simulink library "pwrsys"  (R2018a)
settings: Solver=VariableStepAuto  StartTime=0.0  StopTime=10.0  RelTol=1e-3
values from neighbouring files (symbols this model uses):
  Ts = Ts_c    (= 1e-07)    [PlantStateEquations_abc_Script.m]
undefined symbols (not defined in the file or in its folder): D1, Delta, DiscIntNeverNeededParam, ESS, f_LPF_noise, fn, fsw, grid, gt1, Iap, Kp, PCC, Refmax, Refmin, sim, SIMU, Sn, tctrl, Ti, Ts_control, Ts_PWM, Uabp, Uanp, WT, X, zeta
libraries: $bdroot x71, powerlib x59, powerlib_meascontrol x49, peTransforms x20, PhD_Library x1, sps_avr x1
(part 1 of 4)
settings Model: Creator=daniemot  LastModifiedBy=ericfa

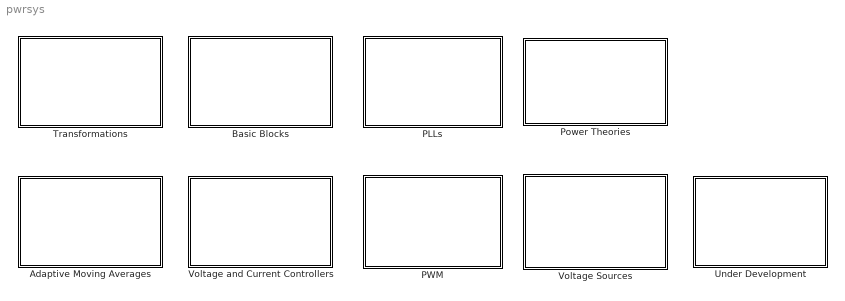
== system pwrsys ==
  Adaptive Moving Averages : Subsystem
  Basic Blocks : Subsystem
  PLLs : Subsystem
  PWM : Subsystem
  Power Theories : Subsystem
  Transformations : Subsystem
  Under Development : Subsystem
  Voltage Sources : Subsystem
  Voltage and Current Controllers : Subsystem

== system pwrsys/Adaptive Moving Averages ==
  AMA with insertion pointer driven buffer : Subsystem  TreatAsAtomicUnit=on  SystemSampleTime=Ts  mask(AMA with insertion pointer driven){NbSize=100, Ts=0.001}
      mask prompts: NbSize "Max number of samples for averaging"; Ts "Sampling time [s]"
      mask help:
      | Adaptive moving average with insertion pointer driven circular buffer
      |
      | Interface
      | Input	x (scalar): signal for averaging
      | 	n (scalar): number of previous samples of the input to be averaged with the current input
      | Output	xavg (scalar): average of the current input and the last n-samples of the input.
      | 	xacc (scalar): internal value sent for accumulation
      | 	xdec (scalar): internal value sent for decumulation
      | Parameters	nmax (scalar): maximum length of the length of the circular buffer
      | 	Ts (scalar): sampling time in [s]
      | Internal circular buffer:
      | 	Insertion pointer: i, always marches forward, x(now) replaces the slot pointed by i
      | 	Retrieval pointer: r, lags i by n samples, zeros the slot once retrieved, allowed to jump backwards, collects all values for decumulation and zeros slots when jumping forward.
      |
      | Prog/rev. semi-history:
      | 	Mota, 2020-11-24: first release
  AMA with lossy buffer : Subsystem  TreatAsAtomicUnit=on  SystemSampleTime=Ts  mask(AMA with a skipping circular buffer.){NbSize=100, Ts=0.001}
      mask prompts: NbSize "Max number of samples for averaging"; Ts "Sampling time [s]"
      mask help:
      | Adaptive moving average built with Matlab's discrete variable time delay
      |
      | Interface
      | Input	x (scalar): signal for averaging
      | 	n (scalar): number of previous samples of the input to be averaged with the current input
      | Output	xavg (scalar): average of the current input and the last n-samples of the input.
      | 	xacc (scalar): internal value sent for accumulation
      | 	xdec (scalar): internal value sent for decumulation
      | Parameters	nmax (scalar): maximum length of the length of the circular buffer
      | 	Ts (scalar): sampling time in [s]
      | Internal circular buffer:
      | 	Matlab's variable discrete time delay
      | 	Skips/double decumulations when n changes
      |
      | Prog/rev. semi-history:
      | 	Mota, 2020-11-24: first release
  AMA with retrieval pointer driven buffer : Subsystem  TreatAsAtomicUnit=on  SystemSampleTime=Ts  mask(AMA with retrieval pointer driven buffer){NbSize=100, Ts=0.001}
      mask prompts: NbSize "Max number of samples for averaging"; Ts "Sampling time [s]"
      mask help:
      | Adaptive moving average with retrieval poitner driven circular buffer
      |
      | Interface
      | Input	x (scalar): signal for averaging
      | 	n (scalar): number of previous samples of the input to be averaged with the current input
      | Output	xavg (scalar): average of the current input and the last n-samples of the input.
      | 	xacc (scalar): internal value sent for accumulation
      | 	xdec (scalar): internal value sent for decumulation
      | Parameters	nmax (scalar): maximum length of the length of the circular buffer
      | 	Ts (scalar): sampling time in [s]
      | Internal circular buffer:
      | 	Retrieval pointer: r, always marches forward, zero the slot after retrieval.
      | 	Insertion pointer: i, marches n slots ahead of r, allowed to jump, sums x(now) to the whichever value present at the insertion slot
      |
      | Prog/rev. semi-history:
      | 	Mota, 2020-11-24: first release
  Subsystem : Subsystem  TreatAsAtomicUnit=on  SystemSampleTime=Ts  mask(HAMA with retrieval pointer driven buffer){NbSize=100, Ts=0.001}
      mask prompts: NbSize "Max number of samples for averaging"; Ts "Sampling time [s]"
      mask help:
      | Hybrid adaptive moving average with three retrieval pointer driven circular buffers.
      |
      | Interface
      | Input	x (scalar): signal for averaging
      | 	n (scalar): number of previous samples of the input to be averaged with the current input
      | Output	xavg (scalar): average of the current input and the last hybrid number of 'n'-samples of the input.
      | 	xavground (scalar): average of the current input and the last round(n)-samples of the input.
      | 	xavgceil (scalar): average of the current input and the last ceil(n)-samples of the input.
      | 	xavgfloor (scalar): average of the current input and the last floor(n)-samples of the input.
      | 	xavgweighed (scalar): average of the current input and the last weighted(n)-samples of the input.
      | Parameters	nmax (scalar): maximum length of the length of the circular buffer
      | 	Ts (scalar): sampling time in [s]
      |
      | Prog/rev. semi-history:
      | 	Mota, 2020-12-08: first release
  WAMA with insertion pointer driven buffer : Subsystem  TreatAsAtomicUnit=on  SystemSampleTime=Ts  mask(WAMA with insertion pointer driven buffer){NbSize=0, Ts=0}
      mask prompts: NbSize "Max number of samples for averaging"; Ts "Sampling time [s]"
      mask help:
      | Adaptive moving average with two insertion pointer driven circular buffers.
      |
      | Interface
      | Input	x (scalar): signal for averaging
      | 	n (scalar): number of previous samples of the input to be averaged with the current input
      | Output	xavg (scalar): weigthed average of the current input and the last 'n'-samples of the input.
      | 	xavgceil (scalar): average of the current input and the last ceil(n)-samples of the input.
      | 	xavgfloor (scalar): average of the current input and the last floor(n)-samples of the input.
      | Parameters	nmax (scalar): maximum length of the length of the circular buffer
      | 	Ts (scalar): sampling time in [s]
      |
      | Prog/rev. semi-history:
      | 	Mota, 2020-11-24: first release
  WAMA with retrieval pointer driven buffers : Subsystem  TreatAsAtomicUnit=on  SystemSampleTime=Ts  mask(WAMA with retrieval pointer driven buffer){NbSize=100, Ts=0.001}
      mask prompts: NbSize "Max number of samples for averaging"; Ts "Sampling time [s]"
      mask help:
      | Adaptive moving average with two retrieval pointer driven circular buffers.
      |
      | Interface
      | Input	x (scalar): signal for averaging
      | 	n (scalar): number of previous samples of the input to be averaged with the current input
      | Output	xavg (scalar): weigthed average of the current input and the last 'n'-samples of the input.
      | 	xavgceil (scalar): average of the current input and the last ceil(n)-samples of the input.
      | 	xavgfloor (scalar): average of the current input and the last floor(n)-samples of the input.
      | Parameters	nmax (scalar): maximum length of the length of the circular buffer
      | 	Ts (scalar): sampling time in [s]
      |
      | Prog/rev. semi-history:
      | 	Mota, 2020-11-24: first release

== system pwrsys/Basic Blocks ==
  DSC : Subsystem
  "DSC Power " : Subsystem
  Digital first order LPF : Subsystem  mask(Digital first-order low-pass filter){Ts=tctrl, fcutout=fn/2^0.5}
      mask prompts: Ts "Sample times [s]"; fcutout "Cutout frequency [Hz]"
      mask help:
      | Continuous time transfer function:  1/(1 + s T)
      | 	where T [s] = 1 / (2 pi fcutout [Hz]).
      |
      | Actual digital transfer function:   alpha / (1 + ( alpha -1) z^{-1} )
      | 	with eq. of diffs.: y = alpha x + (1 - alpha) y z^{-1}
      | 	where alpha = Ts / ( 1/(2 pi fcutout) + Ts)
      mask Display: fprintf('1/(1+sT)');
  Droop controller : Subsystem  mask(Droop controller){Refmax=1, Refmin=-1, Ts=-1, Kp=1, Kd=0, Tr=0.1, flp=100, DB=0}
      mask prompts: Refmax "Max reference"; Refmin "Min reference"; Ts "Sample time"; Kp "Permanent gain"; Kd "Transient gain"; Tr "Reset time [s]"; flp "Low-pass filter cut-off frequency [Hz]"; DB "Dead-band"
      mask help:
      | This block implements a droop controller, i.e. it provides compensation of the input Ref based on the input Delta and Comp.
      |
      | The input Delta is used as input of a PD controller which provides permanent (proportional) and transient (derivative) droop of the input Ref.
      |
      | The input Comp divides the output value of the droop controller and may be used for other types of compensation.
      mask DialogControl DescGroupVar Prompt: Active Power and Frequency Controller
      mask DialogControl DescTextVar Prompt: This block implements a simplified model for power control with droop influence. It can be used either for active power with frequency droop influence or reactive power with voltage droop influence.
      mask DialogControl droop Prompt: Droop control
      mask DialogControl meas Prompt: Delta
  PI controller with Hold : Subsystem  mask(PI controller with anti-windup){Kp=1, Ki=0, Max=1, Min=-1, x0=0, Ts=1e-4}
      mask prompts: Kp "Proportional gain"; Ki "Integral gain"; Max "Maximum output"; Min "Minimum output"; x0 "Initial condition"; Ts "Sampling time"
      mask help:
      | This block implements a PI controller with anti-windup
      |
      | The input hold freezes the integrator and allows implementing anti-windup in control loops with feed-forward or dynamic limits
  PI_Kg_Kp_Ti_AntiWindup : Subsystem  TreatAsAtomicUnit=on  SystemSampleTime=Ts  mask(PI regulator with anti-windup){Ts=0.001, Kg=1, Kp=1, Ti=1, PI_max=1, PI_min=-1}
      mask prompts: Ts "Sampling time [s]"; Kg "Loop gain: Kg [pu]"; Kp "Proportional gain: Kp [pu]"; Ti "Integral time: Ti [s]"; PI_max "Maximum output [pu]"; PI_min "Minimum output [pu]"
      mask help:
      | Discrete PI regulator with forward Euler approximation for the integrator.
      |
      | Transfer function:
      | 	Kg (Kp + 1/sTi)
      |
      | The anti-windup freezes the integrator if the unlimited output of the PI goes beyond the limits.
      |
      | It is possible to disable the proportional (Kp) contribution.
      mask Display: fprintf('Kg(Kp+1/(sTi))');
  PI_Kp_Ti_AntiWindup : Subsystem  TreatAsAtomicUnit=on  SystemSampleTime=Ts  mask(PI regulator with anti-windup){Ts=0.001, Kp=10, Ti=1, PI_max=1, PI_min=-1}
      mask prompts: Ts "Sampling time [s]"; Kp "Proportional gain: Kp [pu]"; Ti "Integral time: Ti [s]"; PI_max "Maximum output [pu]"; PI_min "Minimum output [pu]"
      mask help:
      | Discrete PI regulator with forward Euler approximation for the integrator.
      |
      | Transfer function:
      | 	Kp (1 + sTi) / (sTi)
      |
      | The anti-windup freezes the integrator if the unlimited output of the PI goes beyond the limits.
      mask Display: fprintf('Kp(1+1/(sTi))');
  PQVI : Subsystem  mask(u i p q transducer - No zero sequence){Sn=Sn, Uanp=Uanp, Iap=Iap}
      mask prompts: Sn "Rated three-phase apparent power [VA]"; Uanp "Rated peak phase-to-groud voltage [V]"; Iap "Rated peak line current [A]"
      mask help:
      | Loosely based on Akagi 1984, but with Clarke Transformation for both the current and voltage
      | 	v  = (valpha^2 + vbeta^2)^0.5 / V_phase_peak
      | 	i   = (ialpha^2 + ibeta^2)^0.5 / I_line_peak
      | 	p  = 3/2 * (valpha ialpha +vbeta ibeta) / Sn
      | 	q  = 3/2 * (-valpha ibeta +vbeta ialpha) / Sn
  digital_integrator : Subsystem  SystemSampleTime=Ts  mask(Digital integrator){Ts=tctrl}
      mask prompts: Ts "Sample times [s]"
      mask Display: fprintf('1/s');
  digital_ramp_gen : Subsystem  SystemSampleTime=Ts  mask(Digital ramp generator){Ts=tctrl}
      mask prompts: Ts "Sample times [s]"
      mask help: Allways starts at zero. Can be forced to a value, and will stay there, but in the first two cycles will stay at zero.
      mask Display: fprintf('Ramp');
  pqui_Transd_DSC : Subsystem  mask(DSC u i p q transducer - No zero sequence){Ts=0.000005, fn=50, Sn=Sn, Uanp=Uanp, Iap=Iap}
      mask prompts: Ts "Sampling time [s]"; fn "Rated frequency [Hz]"; Sn "Rated three-phase apparent power [VA]"; Uanp "Rated peak phase-to-groud voltage [V]"; Iap "Rated peak line current [A]"
      mask help:
      | Loosely based on Akagi 1984, but with Clarke Transformation for both the current and voltage
      | 	v  = (valpha^2 + vbeta^2)^0.5 / V_phase_peak
      | 	i   = (ialpha^2 + ibeta^2)^0.5 / I_line_peak
      | 	p  = 3/2 * (valpha ialpha +vbeta ibeta) / Sn
      | 	q  = 3/2 * (-valpha ibeta +vbeta ialpha) / Sn
  pqui_Transd_NoZeroSeq : Subsystem  mask(u i p q transducer - No zero sequence){Sn=Sn, Uanp=Uanp, Iap=Iap}
      mask prompts: Sn "Rated three-phase apparent power [VA]"; Uanp "Rated peak phase-to-groud voltage [V]"; Iap "Rated peak line current [A]"
      mask help:
      | Loosely based on Akagi 1984, but with Clarke Transformation for both the current and voltage
      | 	v  = (valpha^2 + vbeta^2)^0.5 / V_phase_peak
      | 	i   = (ialpha^2 + ibeta^2)^0.5 / I_line_peak
      | 	p  = 3/2 * (valpha ialpha +vbeta ibeta) / Sn
      | 	q  = 3/2 * (-valpha ibeta +vbeta ialpha) / Sn
  pqui_Transd_NoZeroSeq_Filter : Subsystem  mask(u i p q transducer - No zero sequence){Ts=0.001, Sn=1000, fn=50, Uanp=1000, Iap=1000, fcutoutvi=1000, fcutoutpq=1000, zeta=0.7}
      mask prompts: Ts "Sampling time [s]"; Sn "Rated three-phase apparent power [VA]"; fn "Rated frequency [Hz]"; Uanp "Rated peak phase-to-groud voltage [V]"; Iap "Rated peak line current [A]"; fcutoutvi "Cutout freq. low-pass for v&i meas. [Hz]"; fcutoutpq "Cutout freq. low-pass for p&q meas. [Hz]"; zeta "Zeta for all second order filters"
      mask help:
      | Loosely based on Akagi 1984, but with Clarke Transformation for both the current and voltage
      | 	v  = (valpha^2 + vbeta^2)^0.5 / V_phase_peak
      | 	i   = (ialpha^2 + ibeta^2)^0.5 / I_line_peak
      | 	p  = 3/2 * (valpha ialpha +vbeta ibeta) / Sn
      | 	q  = 3/2 * (-valpha ibeta +vbeta ialpha) / Sn
      |
      | Second order low-pass filter for all measurements
      |
      | Notch filter at the rated frequency

== system pwrsys/PLLs ==
  PLL : Subsystem  mask(Matlabs PLL with POS and NEG omega t output){fn=0, Ts=0.00005, Kp_pll=90, Ki_pll=1600, Kd_pll=0, PLL_ini=0}
      mask prompts: fn "Rated frequency [Hz]"; Ts "Sampling time [s]"; Kp_pll "Proportional gain: Kp_pll"; Ki_pll "Integral gain: Ki_pll"; Kd_pll "Derivative gain: Kd_pll"; PLL_ini "PLL initial angle: PLL_ini [degrees]"
  PLL 3-phase abc : Subsystem  mask(3-Phase PLL in the abc frame){fnom=50, fdev=20, zeta=0.707, Kp=100, Ki=50, Kd=1e4, Tr=100, Ts=1e-4, wt0=0}
      mask prompts: fnom "Rated frequency [Hz]"; fdev "Maximum frequency deviation [Hz]"; zeta "Damping ratio"; Kp "Proportional gain"; Ki "Integral gain"; Kd "Derivative gain"; Tr "Reset time [s]"; Ts "Sampling time [s]"; wt0 "Initial angle [rad/s]"
      mask help: This block implements a 3-phase PLL in the abc reference frame.
      mask init:
      | wn = fnom/(4*zeta);
      mask DialogControl freqFilter Prompt: Frequency filter
      mask DialogControl ctrl Prompt: Controller
  PLL_pu : Subsystem  mask(Matlabs PLL with POS and NEG omega t output){fn=0, Ts=0.00005, Kp_pll=90, Ki_pll=1600, Kd_pll=0, PLL_ini=0}
      mask prompts: fn "Rated frequency [Hz]"; Ts "Sampling time [s]"; Kp_pll "Proportional gain: Kp_pll"; Ki_pll "Integral gain: Ki_pll"; Kd_pll "Derivative gain: Kd_pll"; PLL_ini "PLL initial angle: PLL_ini [degrees]"

== system pwrsys/PWM ==
  PWM_abc_negwt_acb : Subsystem  mask(Scaling of vdq ref and PWM gate generation){fsw=50, Ts=1/200000, Uabp=1000, PWM_Ini_Phase=90}
      mask prompts: fsw "Switching frequency [Hz]"; Ts "Sampling time [s]"; Uabp "Rated peak line voltage [V]"; PWM_Ini_Phase "PWM carrier initial phase [degrees]"
      mask help:
      | Scales vdq_ref by: U_line_peak / Udc
      |
      | Add third harmonic to uabc_ref for overmodulation
  PWM_single_dual : Subsystem  mask(Scaling of vdq ref and PWM gate generation){fsw=50, Ts=1/200000, Uabp=1000, PWM_Ini_Phase=90}
      mask prompts: fsw "Switching frequency [Hz]"; Ts "Sampling time [s]"; Uabp "Rated peak line voltage [V]"; PWM_Ini_Phase "PWM carrier initial phase [degrees]"
      mask help:
      | Scales vdq_ref by: U_line_peak / Udc
      |
      | Add third harmonic to uabc_ref for overmodulation

== system pwrsys/Power Theories ==
  note: CPT Single Phase
  Instantaneous Power xyz : Subsystem  mask(Instantaneous Power xyz){typeTransf=Amplitude-invariant}
      mask prompts: typeTransf "Type of transformation"
      mask init:
      | switch typeTransf
      |     case 1
      |         a = 1;
      |         b = 1;
      |     case 2
      |         a = 1.5;
      |         b = 3;
      | end
      mask TypeOptions typeTransf: Amplitude-invariant | Power-invariant
  Single phase CPT Lossy AMA : Subsystem  TreatAsAtomicUnit=on  SystemSampleTime=Ts  mask(Single phase CPT transducer with Skipping AMAs){NbSize=100, Ts=0.001}
      mask prompts: NbSize "Maximum number of samples per period"; Ts "Sampling time [s]"
      mask help:
      | Input	Voltage: v, scalar
      | 	Current: i, scalar
      | 	Frequecy: f, scalar in [Hz]
      | Output	Active power: p
      | 	Active current: ia
      | 	Reactive power: q
      | 	Reactive energy: w
      | 	Reactive current: ir
      | 	Void current: iv
      | 	Integral of the voltage: vint
      | 	Bias of the int. of the volt.: vintbias
      | 	Voltage times current: vi
      | 	Unbiased int. voltage times current: vinthati
      | Parameters	nmax (scalar): maximum length of the length of the circular buffers
      | 	Ts (scalar): sampling time in [s]
      |
      | Prog/rev. semi-history:
      | 	Mota, 2020-11-24: first release
      | 	Mota, 2020-12-08: added voltages and currents to interface
  Single phase CPT Retrieval AMA : Subsystem  TreatAsAtomicUnit=on  SystemSampleTime=Ts  mask(Single Phase CPT Retrieval AMAs){NbSize=100, Ts=0.001}
      mask prompts: NbSize "Maximum number of samples per period"; Ts "Sampling time [s]"
      mask help:
      | Input	Voltage: v, scalar
      | 	Current: i, scalar
      | 	Frequecy: f, scalar in [Hz]
      | Output	Active power: p
      | 	Active current: ia
      | 	Reactive power: q
      | 	Reactive energy: w
      | 	Reactive current: ir
      | 	Void current: iv
      | 	Integral of the voltage: vint
      | 	Bias of the int. of the volt.: vintbias
      | 	Voltage times current: vi
      | 	Unbiased int. voltage times current: vinthati
      | Parameters	nmax (scalar): maximum length of the length of the circular buffers
      | 	Ts (scalar): sampling time in [s]
      |
      | Prog/rev. semi-history:
      | 	Mota, 2020-11-24: first release
      | 	Mota, 2020-12-08: added voltages and currents to interface
  Single phase CPT Retrieval HAMA : Subsystem  TreatAsAtomicUnit=on  SystemSampleTime=Ts  mask{NbSize=100, Ts=0.001}
      mask prompts: NbSize "Maximum number of samples per period"; Ts "Sampling time [s]"
      mask help:
      | Input	Voltage: v, scalar
      | 	Current: i, scalar
      | 	Frequecy: f, scalar in [Hz]
      | Output	Active power: p
      | 	Active current: ia
      | 	Reactive power: q
      | 	Reactive energy: w
      | 	Reactive current: ir
      | 	Void current: iv
      | 	Integral of the voltage: vint
      | 	Bias of the int. of the volt.: vintbias
      | 	Voltage times current: vi
      | 	Unbiased int. voltage times current: vinthati
      | Parameters	nmax (scalar): maximum length of the length of the circular buffers
      | 	Ts (scalar): sampling time in [s]
      |
      | Prog/rev. semi-history:
      | 	Mota, 2020-12-08: first release
  Single phase CPT Retrieval WAMA : Subsystem  TreatAsAtomicUnit=on  SystemSampleTime=Ts  mask(Single phase CPT with Retrieval WAMAs){NbSize=100, Ts=0.001}
      mask prompts: NbSize "Maximum number of samples per period"; Ts "Sampling time [s]"
      mask help:
      | Input	Voltage: v, scalar
      | 	Current: i, scalar
      | 	Frequecy: f, scalar in [Hz]
      | Output	Active power: p
      | 	Active current: ia
      | 	Reactive power: q
      | 	Reactive energy: w
      | 	Reactive current: ir
      | 	Void current: iv
      | 	Integral of the voltage: vint
      | 	Bias of the int. of the volt.: vintbias
      | 	Voltage times current: vi
      | 	Unbiased int. voltage times current: vinthati
      | Parameters	nmax (scalar): maximum length of the length of the circular buffers
      | 	Ts (scalar): sampling time in [s]
      |
      | Prog/rev. semi-history:
      | 	Mota, 2020-11-24: first release
      | 	Mota, 2020-12-08: added voltages and currents to interface

== system pwrsys/Transformations ==
  note: Foundation
  note: ABC -> DQ
  abc to xyz : Subsystem  mask(Clarke transformation){typeTransf=Amplitude-invariant}
      mask prompts: typeTransf "Type of transformation"
      mask init:
      | switch typeTransf
      |     case 1
      |         a = 1/3;
      |         b = 1/sqrt(3);
      |         c = sqrt(2)/3;
      |     case 2
      |         a = 1/sqrt(6);
      |         b = 1/sqrt(2);
      |         c = 1/sqrt(3);
      | end
      mask TypeOptions typeTransf: Amplitude-invariant | Power-invariant
  abc-dq_DDSRF_PLL_Based : Subsystem  mask(abc -> dq based on DDSRF PLL){Ts=Ts_control, fc=fn/2^0.5}
      mask prompts: Ts "Sampling time [s]"; fc "Cutout freq. low pass [Hz]"
      mask help:
      | abc -> dq transducer based on the Decoupled Double Synchronous Reference Frame PLL for Power Converters Control from Rodriguez 2007.
      | The PLL is not implemented, but an output with eq is available for using in a PLL
  abc_dq : Subsystem  mask(abc->dq with Matlab){Ts=0.001, fn=100, fcutoutv=1000, fcutouti=1000, zeta=0.707}
      mask prompts: Ts "Sampling time [s]"; fn "Notch frequency [Hz]"; fcutoutv "Cutout freq. low-pass for vdq meas. [Hz]"; fcutouti "Cutout freq. low-pass for idq meas. [Hz]"; zeta "Zeta for notch filters"
  abc_dq_bypassnotch : Subsystem  mask(abc->dq with Matlab){Ts=0.001, fn=100, fcutoutv=1000, fcutouti=1000, zeta=0.707}
      mask prompts: Ts "Sampling time [s]"; fn "Notch frequency [Hz]"; fcutoutv "Cutout freq. low-pass for vdq meas. [Hz]"; fcutouti "Cutout freq. low-pass for idq meas. [Hz]"; zeta "Zeta for notch filters"
      mask help:
      | To be done
      |
      | Max buffer size for DSC 500 samples
  abc_dq_single_notch_dsc : Subsystem  mask(abc->dq with Matlab){Ts=0.001, fn=100, zeta=0.707}
      mask prompts: Ts "Sampling time [s]"; fn "Notch frequency [Hz]"; zeta "Zeta for notch filters"
      mask help:
      | To be done
      |
      | Max buffer size for DSC 500 samples
  abc_dq_with_AMA : Subsystem  mask(abc->dq with Matlab){Ts=0.001, fn=100, fmin=0, fmax=0, fcutoutv=1000, fcutouti=1000}
      mask prompts: Ts "Sampling time [s]"; fn "Rated grid frequency [Hz]"; fmin "Min. acceptable grid freq [Hz]"; fmax "Max. acceptable grid freq [Hz]"; fcutoutv "Cutout freq. low-pass for vdq meas. [Hz]"; fcutouti "Cutout freq. low-pass for idq meas. [Hz]"
  dqz to xyz : Subsystem  mask(Inverse Park transformation){}
  xyz to abc : Subsystem  mask(Inverse Clarke transformation){typeTransf=Amplitude-invariant}
      mask prompts: typeTransf "Type of transformation"
      mask init:
      | switch typeTransf
      |     case 1
      |         a = 1;
      |         b = sqrt(3)/2;
      |         c = 1/2;
      |         d = 1/sqrt(2);
      |     case 2
      |         a = sqrt(2/3);
      |         b = 1/sqrt(2);
      |         c = 1/sqrt(6);
      |         d = 1/sqrt(3);
      | end
      mask TypeOptions typeTransf: Amplitude-invariant | Power-invariant
  xyz to dqz : Subsystem  mask(Inverse Park transformation){}

== system pwrsys/Under Development ==

== system pwrsys/Voltage Sources ==
  Balanced_3_phase_Vsource : Subsystem  mask(Three-phase ideal voltage source){BaseAmp=1, fn=50}
      mask prompts: BaseAmp "Base phase-to-neutral amplitude [V]"; fn "Base frequency [Hz]"
      mask help:
      | Three-phase balanced ideal voltage source with neutral point not connected.
      | The voltage source can be connected in series with others.
      |
      | va [V] = amp_pu*BaseAmp*sin(2*pi*f_pu*fn*time + phase_deg*pi/180)
      | vb [V] = amp_pu*BaseAmp*sin(2*pi*f_pu*fn*time + phase_deg*pi/180 + Ph_b_sign*2*pi/3)
      | vc [V] = amp_pu*BaseAmp*sin(2*pi*f_pu*fn*time + phase_deg*pi/180 + Ph_c_sign*2*pi/3)
      |
      | If Pos1_Neg-1 = 1
      | 	Ph_b_sign = -1
      | 	Ph_c_sign = +1
      |
      | If Pos1_Neg-1 = -1
      | 	Ph_b_sign = +1
      | 	Ph_c_sign = -1
  DCL_LSC_LCL_Trafo_NoSwitching : Subsystem  mask(DCL + LSC + LCL + Trafo){Sn=WT.Sb, fn=fn, Uhv_ab=WT.ColSys.Ub, Uab=WT.LSC.Ub, lf2=WT.LSC.lf2, rf2=WT.LSC.rf2, Lf1=WT.LSC.Lf1, Rf1=WT.LSC.Rf1, Cf=WT.LSC.Cf, Rc=WT.LSC.Rc, Cdc=WT.LSC.Cf, Udc0=WT.LSC.Cf, Tsm=WT.LSC.Rc, Tstart=WT.LSC.Rc}
      mask prompts: Sn "Rated apparent power [VA]"; fn "Rated frequency [Hz]"; Uhv_ab "Trafo HV rated line voltage [V]"; Uab "Trafo LV rated line voltage [V]"; lf2 "Trafo short-circuit inductance, lf2 [pu]"; rf2 "Trafo short-circuit resistance, rf2 [pu]"; Lf1 "Inverter side inductande, Lf1 [H]"; Rf1 "Inverter side parasitic resistance, Rf1 [Ohm]"; Cf "Shunt branch capacitance, Cf [F]"; Rc "Shunt branch damping resistance, Rc [Ohm]"; Cdc "DC-link shunt capacitance, Cdc [F]"; Udc0 "DC-link initial voltage [V]"; Tsm "Measurement sampling time [s]"; Tstart "Start time [s]"
      mask help:
      | DC Link + Line-side converter + LCL filter + Transformer
      |
      | DCL: current sources
      | 	Cdc: shunt capacitor of DC-link
      |
      | LSC: voltage source
      | 	fpwm: PWM frequency
      | LCL:
      | 	Lf1 + Rf1: inverter side reactor
      | 	Cf + Rc: shunt capacitor and damping resistor
      | 	Lf2 + Rf2: transformer short circuit inductance and resistance
      |
      | Transformer:	Y d1
      | 	HV: Y ungrounded
      | 	LV: delta
      |
      | High resistive grounding on LV side of tranformer (0.001W)
  LSC_LCL_Trafo : Subsystem  mask(LSC + LCL + Trafo){Sn=WT.Sb, fn=fn, Uhv_ab=WT.ColSys.Ub, Uab=WT.LSC.Ub, lf2=WT.LSC.lf2, rf2=WT.LSC.rf2, Lf1=WT.LSC.Lf1, Rf1=WT.LSC.Rf1, Cf=WT.LSC.Cf, Rc=WT.LSC.Rc}
      mask prompts: Sn "Rated apparent power [VA]"; fn "Rated frequency [Hz]"; Uhv_ab "Trafo HV rated line voltage [V]"; Uab "Trafo LV rated line voltage [V]"; lf2 "Trafo short-circuit inductance, lf2 [pu]"; rf2 "Trafo short-circuit resistance, rf2 [pu]"; Lf1 "Inverter side inductande, Lf1 [H]"; Rf1 "Inverter side parasitic resistance, Rf1 [Ohm]"; Cf "Shunt branch capacitance, Cf [F]"; Rc "Shunt branch damping resistance, Rc [Ohm]"
      mask help:
      | Line side converter + LCL filter + Transformer
      |
      | LSC: switching devices
      | LCL:
      | 	Lf1 + Rf1: inverter side reactor
      | 	Cf + Rc: shunt capacitor and damping resistor
      | 	Lf2 + Rf2: transformer short circuit inductance and resistance
      |
      | Transformer:	Y d1
      | 	HV: Y ungrounded
      | 	LV: delta
      |
      | High resistive grounding on LV side of tranformer (0.001W)
  LSC_LCL_Trafo_AvgxSwitch : Subsystem  mask(LSC + LCL + Trafo){Sn=WT.Sb, fn=fn, Uhv_ab=WT.ColSys.Ub, Uab=WT.LSC.Ub, lf2=WT.LSC.lf2, rf2=WT.LSC.rf2, Lf1=WT.LSC.Lf1, Rf1=WT.LSC.Rf1, Cf=WT.LSC.Cf, Rc=WT.LSC.Rc}
      mask prompts: Sn "Rated apparent power [VA]"; fn "Rated frequency [Hz]"; Uhv_ab "Trafo HV rated line voltage [V]"; Uab "Trafo LV rated line voltage [V]"; lf2 "Trafo short-circuit inductance, lf2 [pu]"; rf2 "Trafo short-circuit resistance, rf2 [pu]"; Lf1 "Inverter side inductande, Lf1 [H]"; Rf1 "Inverter side parasitic resistance, Rf1 [Ohm]"; Cf "Shunt branch capacitance, Cf [F]"; Rc "Shunt branch damping resistance, Rc [Ohm]"
      mask help:
      | Line side converter + LCL filter + Transformer
      |
      | LSC: switching devices
      | LCL:
      | 	Lf1 + Rf1: inverter side reactor
      | 	Cf + Rc: shunt capacitor and damping resistor
      | 	Lf2 + Rf2: transformer short circuit inductance and resistance
      |
      | Transformer:	Y d1
      | 	HV: Y ungrounded
      | 	LV: delta
      |
      | High resistive grounding on LV side of tranformer (0.001W)
  LSC_LCL_Trafo_NoSwitching : PhD_Library/Offshore_Oil_and_Wind/LSC_LCL_Trafo_NoSwitching  Sn=WT.Sb  fn=fn  Uhv_ab=WT.ColSys.Ub  Uab=WT.LSC.Ub  lf2=WT.LSC.lf2  rf2=WT.LSC.rf2  Lf1=WT.LSC.Lf1  Rf1=WT.LSC.Rf1  Cf=WT.LSC.Cf  Rc=WT.LSC.Rc
  SM_TG_EXC : Subsystem  SystemSampleTime=10*sim.tStep  mask(Synchronous Generator with Governor and Exciter){SMVn=PCC.Un, SMPn=gt1.SM.Sn, SMcosphi=gt1.SM.cosphi, SMfn=PCC.Fn, SMp=gt1.SM.p, SMM=gt1.SM.M, SMXd=gt1.SM.Xd, SMXdp=gt1.SM.Xdp, SMXdpp=gt1.SM.Xdpp, SMXq=gt1.SM.Xq, SMXqpp=gt1.SM.Xqpp, SMXl=gt1.SM.Xl, SMRs=gt1.SM.Rs, SMTdpSC=gt1.SM.TdpSC, SMTdppSC=gt1.SM.TdppSC, SMTqppSC=gt1.SM.TqppSC, TurbT=gt1.Turb.T, GovKp=gt1.P.Kp, GovKd=gt1.P.Kd, GovTr=gt1.P.Tr, GovFlp=gt1.P.flp, GovDB=gt1.P.DB, ExcTr=gt1.exc.Tr, ExcKa=gt1.exc.Ka, ExcVRMax=gt1.exc.VRmax, ExcVRMin=gt1.exc.VRmin, ExcKf=gt1.exc.Kf, ExcTf=gt1.exc.Tf, ExcTb=gt1.exc.Tb, ExcTc=gt1.exc.Tc, ExcTb1=gt1.exc.Tb1, ExcTc1=gt1.exc.Tc1}
      mask prompts: SMVn "Voltage [V]"; SMPn "Apparent power [VA]"; SMcosphi "Power factor"; SMfn "Frequency [Hz]"; SMp "Pairs of poles"; SMM "Inertia constant [s]"; SMXd "d-axis steady-state"; SMXdp "d-axis transient"; SMXdpp "d-axis subtransient"; SMXq "q-axis steady-state"; SMXqpp "q-axis subtransient"; SMXl "Leakage"; SMRs "Stator (armature) resistance"; SMTdpSC "d-axis transient time"; SMTdppSC "d-axis subtransient time"; SMTqppSC "q-axis subtransient time"; TurbT "Equivalent first-order delay [s]"; GovKp "Permanent droop (primary control)"; GovKd "Transient droop (primary control)"; GovTr "Reset time transient droop (primary control)"; GovFlp "Low-pass frequency [Hz]"; GovDB "Deadband [pu]"; ExcTr "Input filter time constant [s]"; ExcKa "Proportional gain"; ExcVRMax "Maximum output [pu]"; ExcVRMin "Minimum output [pu]"; ExcKf "Rate feedback (derivative) gain"; ExcTf "Rate feedback (reset) time [s]"; ExcTb "1st lag time constant [s]"; ExcTc "1st lead time constant [s]"; ExcTb1 "2nd lag time constant [s]"; ExcTc1 "2nd lead time constant [s]"
      mask help:
      | Synchronous machine + Generic Turbine Governor + IEEE ST1A Exciter
      |
      | This block is built using elements of the Simscape Specialized Power Systems library.
      |
      | Inputs:
      | Psp - Active power (P) setpoint in pu.
      |     Feed-forwarded to the turbine governor's Pxf droop controller. For precise P control, implement an external P controller.
      |
      | Vsp - RMS average voltage in pu.
      |     Connected to the Vref input of the IEEE ST1A Exciter.
      |
      | PSS - PSS contribution in pu.
      |     Connected to the Vstab input of the IEEE ST1A Exciter. Implement the PSS control loop externally.
      mask DialogControl ParameterGroupVar Prompt: Synchronous Machine
      mask DialogControl Container11_copy Prompt: Rated values
      mask DialogControl Container11 Prompt: Impedances [pu]
      mask DialogControl Container19 Prompt: Short-circuit time constants [s]
      mask DialogControl Container3 Prompt: Turbine
      mask DialogControl Container4 Prompt: Controllers
      mask DialogControl Container6 Prompt: Governor
      mask DialogControl Container8 Prompt: Exciter

== system pwrsys/Voltage and Current Controllers ==
  DualRegulator : Subsystem  mask(Notch based dual dq current regulator){Ts=Ts_control, fgrid=fn, fcutoutLPF=f_LPF_noise, zetanotch=zeta, PI_Kp=Kp, PI_Ti=Ti, PI_X=X, PI_max=1.5, PI_min=-1.5, PWM_Ts=Ts_PWM, PWM_fsw=fsw, PWM_Uabp=Uabp, PWM_Ini=90}
      mask prompts: Ts "Sampling time controller [s]"; fgrid "Grid frequency [Hz]"; fcutoutLPF "Cutout frequency low pass filters [Hz]"; zetanotch "Damping notch filters"; PI_Kp "Proportional gain Kp [pu/pu]"; PI_Ti "Integrator time Ti [s]"; PI_X "Decoupling reactance X [pu]"; PI_max "PI max [pu]"; PI_min "PI min [pu]"; PWM_Ts "Sampling time PWM [s]"; PWM_fsw "Switching frequency [Hz]"; PWM_Uabp "Rated peak line voltage [V]"; PWM_Ini "Initial phase of carrier [degrees]"
      mask help: To be used with "abc -> dq" and "acb -> dq" transformations. When va = V sin (wt), vb = V sin (wt-120), vc = V sin (wt+120), -> vd = V vq=0.
      mask DialogControl Container2 Prompt: Transducers
      mask DialogControl Container7 Prompt: PI regulator
      mask DialogControl Container5 Prompt: PWM
  Idq_Dec_Signs_Fdbk_Ref : Subsystem  mask(Idq Controller - PI regulator with anti-windup){Ts=Ts_control, fn=50, Kp=0.4, Ti=0.13, L=0.3, PI_max=1.5, PI_min=-1.5, TrafoPhaseComp=0}
      mask prompts: Ts "Sampling time [s]"; fn "Rated frequency: fn [Hz]"; Kp "Proportional gain: Kp [pu]"; Ti "Integral time: Ti [s]"; L "DQ decoupl. inductance: L [pu]"; PI_max "Maximum output [pu]"; PI_min "Minimum output [pu]"; TrafoPhaseComp "Transformer phase compensation [rad]"
      mask help:
      | Idq Controller
      | Discrete PI regulator with forward Euler approximation for the integrator.
      | Transfer function: 	Kp (1 + sTi) / (sTi)
      | The anti-windup freezes the integrator if the unlimited output of the PI goes beyond the limits.
      |
      | Phase compensation for transformer winding: PhaseTrafoComp
  Single_Dual_Current_Regulator : Subsystem  mask(Notch based dual dq current regulator){Ts=Ts_control, fgrid=fn, zetanotch=zeta, PI_Kp=Kp, PI_Ti=Ti, PI_X=X, PI_max=1.5, PI_min=-1.5, PWM_Ts=Ts_PWM, PWM_fsw=fsw, PWM_Uabp=Uabp, PWM_Ini=90}
      mask prompts: Ts "Sampling time controller [s]"; fgrid "Grid frequency [Hz]"; zetanotch "Damping notch filters"; PI_Kp "Proportional gain Kp [pu/pu]"; PI_Ti "Integrator time Ti [s]"; PI_X "Decoupling reactance X [pu]"; PI_max "PI max [pu]"; PI_min "PI min [pu]"; PWM_Ts "Sampling time PWM [s]"; PWM_fsw "Switching frequency [Hz]"; PWM_Uabp "Rated peak line voltage [V]"; PWM_Ini "Initial phase of carrier [degrees]"
      mask help: To be used with "abc -> dq" and "acb -> dq" transformations. When va = V sin (wt), vb = V sin (wt-120), vc = V sin (wt+120), -> vd = V vq=0.
      mask DialogControl Container2 Prompt: Transducers
      mask DialogControl Container7 Prompt: PI regulator
      mask DialogControl Container5 Prompt: PWM
  Uac_Controller : Subsystem  mask(Udc Controller - PI regulator with anti-windup){Ts=Ts_control, Kg=1, Kp=WT.LSC.Kp, Ti=WT.LSC.Ti, PI_max=1.5, PI_min=-1.5}
      mask prompts: Ts "Sampling time [s]"; Kg "Loop gain: Kg [pu]"; Kp "Proportional gain: Kp [pu]"; Ti "Integral time: Ti [s]"; PI_max "Maximum output [pu]"; PI_min "Minimum output [pu]"
      mask help:
      | Udc Controller
      | Discrete PI regulator with forward Euler approximation for the integrator.
      | Transfer function: 	Kp (1 + sTi) / (sTi)
      | The anti-windup freezes the integrator if the unlimited output of the PI goes beyond the limits.
  Udc_Controller : Subsystem  mask(Udc Controller - PI regulator with anti-windup){Ts=Ts_control, Kp=WT.LSC.Kp, Ti=WT.LSC.Ti, PI_max=1.5, PI_min=-1.5}
      mask prompts: Ts "Sampling time [s]"; Kp "Proportional gain: Kp [pu]"; Ti "Integral time: Ti [s]"; PI_max "Maximum output [pu]"; PI_min "Minimum output [pu]"
      mask help:
      | Udc Controller
      | Discrete PI regulator with forward Euler approximation for the integrator.
      | Transfer function: 	Kp (1 + sTi) / (sTi)
      | The anti-windup freezes the integrator if the unlimited output of the PI goes beyond the limits.
  idqref_gen_for_cnst_p : Subsystem  mask(idq reference gen for neg. seq. controller){Ts_control=Ts_control}
      mask prompts: Ts_control "Sampling time [s]"
      mask help:
      | Calculation of the negative sequence references for removing active power second harmonic oscillations.
      | Reactive power is allowed to oscillated with second harmonic.
      |
      | To be used with "abc -> dq" and "acb -> dq" transformations. When va = V sin (wt), vb = V sin (wt-120), vc = V sin (wt+120), -> vd = V vq=0.
      |
      | In "expanded" matrix form
      | | idn | = - | -vdp  +vqp |^{-1} * | -vdn  +vqn | * | idp |
      | | iqn | =   | +vqp  +vdp |        | -vdn  +vqn |   | idq |
      | In matrix form
      | idqn  = - vdqp^{-1} * vdqn * idqp
      |
      | Not tested for "abc (-omega) -> dq" (which I think is the formulation of Chaudhary 2012.
      | Derived independently from, but later noticed that it was proposed by Chaudhary in 2012 at "Negative Sequence Current Control in Wind Power Plants With VSC-HVDC Connection", check eq. (11).

== system pwrsys/Adaptive Moving Averages/AMA with insertion pointer driven buffer ==
  In1 : Inport
  In2 : Inport  Port=2
  Constant3 : Constant  Value=NbSize
  MATLAB Function : MATLAB Function  TreatAsAtomicUnit=on
  Out1 : Outport
  Out2 : Outport  Port=2
  Out3 : Outport  Port=3
  wires:
  In2/1 -> MATLAB Function/2(n)  "n"
  MATLAB Function/1(xavg) -> Out1/1  "xavg"
  Constant3/1 -> MATLAB Function/3(Nb)
  MATLAB Function/2(xacc) -> Out2/1  "xacc"
  MATLAB Function/3(xdec) -> Out3/1  "xdec"
  In1/1 -> MATLAB Function/1(x)  "x"

== system pwrsys/Adaptive Moving Averages/AMA with lossy buffer ==
  x : Inport
  n : Inport  Port=2
  Add1 : Sum
  Add4 : Sum  Inputs=+-
  Constant : Constant
  Delay2 : Delay  DelayLength=1  InitialCondition=0  UseCircularBuffer=on  SampleTime=Ts
  Divide1 : Product  Inputs=*/
  Max : MinMax  Function=max  Inputs=2
  Rounding Function : Rounding  Operator=round
  Variable Integer Delay2 : Delay  DelayLengthSource=Input port  DelayLengthUpperLimit=NbSize  UseCircularBuffer=on  SampleTime=Ts
      settings: InputPortMap=u0,p1
  Zero-Order Hold : ZeroOrderHold  Commented=through  SampleTime=Ts
  Zero-Order Hold1 : ZeroOrderHold  Commented=through  SampleTime=Ts
  xavg : Outport
  xacc : Outport  Port=2
  xdec : Outport  Port=3
  wires:
  n/1 -> Zero-Order Hold1/1  "n"
  x/1 -> Zero-Order Hold/1  "x"
  Divide1/1 -> Add4/1, Variable Integer Delay2/1, xacc/1  "xacc"
  Variable Integer Delay2/1 -> Add4/2, xdec/1  "xdec"
  Constant/1 -> Max/2
  Max/1 -> Variable Integer Delay2/2  "n"
  Add4/1 -> Add1/1  "xavg"
  Add1/1 -> Delay2/1, xavg/1  "xavg"
  Delay2/1 -> Add1/2
  Zero-Order Hold/1 -> Divide1/1
  Zero-Order Hold1/1 -> Rounding Function/1
  Rounding Function/1 -> Divide1/2, Max/1

== system pwrsys/Adaptive Moving Averages/AMA with retrieval pointer driven buffer ==
  In1 : Inport
  In2 : Inport  Port=2
  Constant3 : Constant  Value=NbSize
  MATLAB Function : MATLAB Function  TreatAsAtomicUnit=on
  Out1 : Outport
  Out2 : Outport  Port=2
  Out3 : Outport  Port=3
  wires:
  MATLAB Function/3(xdec) -> Out3/1  "xdec"
  MATLAB Function/1(xavg) -> Out1/1  "xavg"
  Constant3/1 -> MATLAB Function/3(Nb)
  In1/1 -> MATLAB Function/1(x)  "x"
  In2/1 -> MATLAB Function/2(n)  "n"
  MATLAB Function/2(xacc) -> Out2/1  "xacc"

== system pwrsys/Adaptive Moving Averages/Subsystem ==
  In1 : Inport
  In2 : Inport  Port=2
  Constant3 : Constant  Value=NbSize
  MATLAB Function : MATLAB Function  TreatAsAtomicUnit=on
  Terminator{,1..3} (4 alike) : Terminator
  Out1 : Outport
  Out3 : Outport  Port=2
  Out4 : Outport  Port=3
  Out2 : Outport  Port=4
  Out5 : Outport  Port=5
  wires:
  MATLAB Function/1(xavg) -> Out1/1  "xavg"
  MATLAB Function/2(xavground) -> Out3/1  "xavground"
  MATLAB Function/3(xavgceil) -> Out4/1  "xavgceil"
  MATLAB Function/4(xavgfloor) -> Out2/1  "xavgfloor"
  MATLAB Function/6(nr) -> Terminator/1  "nr"
  MATLAB Function/7(nf) -> Terminator1/1  "nf"
  MATLAB Function/8(nc) -> Terminator2/1  "nc"
  MATLAB Function/9(changecnt) -> Terminator3/1  "changenc"
  In1/1 -> MATLAB Function/1(x)  "x"
  Constant3/1 -> MATLAB Function/3(Nb)
  In2/1 -> MATLAB Function/2(n)  "n"
  MATLAB Function/5(xavgweigthed) -> Out5/1  "xavgw"

== system pwrsys/Adaptive Moving Averages/WAMA with insertion pointer driven buffer ==
  In1 : Inport
  In2 : Inport  Port=2
  AMA with insertion pointer driven buffer : $bdroot/Adaptive Moving Averages/AMA with insertion pointer driven buffer  NbSize=NbSize  Ts=Ts
  AMA with insertion pointer driven buffer1 : $bdroot/Adaptive Moving Averages/AMA with insertion pointer driven buffer  NbSize=NbSize  Ts=Ts
  Add : Sum
  Constant : Constant
  Constant1 : Constant
  Floor : Rounding  Operator=ceil
  Floor1 : Rounding
  Max : MinMax  Function=max  Inputs=2
  Product : Product
  Product1 : Product
  Subtract : Sum  Inputs=+-
  Subtract1 : Sum  Inputs=+-+
  Terminator{,1..3} (4 alike) : Terminator
  Out1 : Outport
  Out2 : Outport  Port=2
  Out3 : Outport  Port=3
  wires:
  AMA with insertion pointer driven buffer/1 -> Out2/1, Product/1  "xavgceil"
  AMA with insertion pointer driven buffer/2 -> Terminator/1
  Floor1/1 -> AMA with insertion pointer driven buffer1/2, Subtract1/3, Subtract/2
  Product1/1 -> Add/2
  Subtract/1 -> Product/2
  Product/1 -> Add/1
  Add/1 -> Out1/1  "xavg"
  Subtract1/1 -> Product1/1
  AMA with insertion pointer driven buffer1/2 -> Terminator2/1
  AMA with insertion pointer driven buffer1/3 -> Terminator3/1
  Floor/1 -> AMA with insertion pointer driven buffer/2
  AMA with insertion pointer driven buffer1/1 -> Product1/2, Out3/1  "xavgfloor"
  AMA with insertion pointer driven buffer/3 -> Terminator1/1
  Constant1/1 -> Max/2
  Max/1 -> Floor1/1, Subtract1/2, Subtract/1, Floor/1
  In2/1 -> Max/1  "n"
  Constant/1 -> Subtract1/1
  In1/1 -> AMA with insertion pointer driven buffer1/1, AMA with insertion pointer driven buffer/1  "x"

== system pwrsys/Adaptive Moving Averages/WAMA with retrieval pointer driven buffers ==
  In1 : Inport
  In2 : Inport  Port=2
  AMA with retrieval pointer driven buffer : $bdroot/Adaptive Moving Averages/AMA with retrieval pointer driven buffer  NbSize=NbSize  Ts=Ts
  AMA with retrieval pointer driven buffer1 : $bdroot/Adaptive Moving Averages/AMA with retrieval pointer driven buffer  NbSize=NbSize  Ts=Ts
  Add : Sum
  Constant : Constant
  Constant1 : Constant
  Floor : Rounding  Operator=ceil
  Floor1 : Rounding
  Max : MinMax  Function=max  Inputs=2
  Product : Product
  Product1 : Product
  Subtract : Sum  Inputs=+-
  Subtract1 : Sum  Inputs=+-+
  Terminator{,1..3} (4 alike) : Terminator
  Out1 : Outport
  Out2 : Outport  Port=2
  Out3 : Outport  Port=3
  wires:
  AMA with retrieval pointer driven buffer/3 -> Terminator1/1
  In1/1 -> AMA with retrieval pointer driven buffer1/1, AMA with retrieval pointer driven buffer/1  "x"
  Floor1/1 -> AMA with retrieval pointer driven buffer1/2, Subtract1/3, Subtract/2
  AMA with retrieval pointer driven buffer/2 -> Terminator/1
  Product1/1 -> Add/2
  Subtract1/1 -> Product1/1
  Add/1 -> Out1/1  "xavg"
  Product/1 -> Add/1
  Subtract/1 -> Product/2
  AMA with retrieval pointer driven buffer/1 -> Out2/1, Product/1  "xavgceil"
  Floor/1 -> AMA with retrieval pointer driven buffer/2
  In2/1 -> Max/1  "n"
  AMA with retrieval pointer driven buffer1/2 -> Terminator2/1
  Constant/1 -> Subtract1/1
  AMA with retrieval pointer driven buffer1/1 -> Product1/2, Out3/1  "xavgfloor"
  AMA with retrieval pointer driven buffer1/3 -> Terminator3/1
  Constant1/1 -> Max/2
  Max/1 -> Floor1/1, Subtract1/2, Subtract/1, Floor/1

== system pwrsys/Basic Blocks/DSC ==
  note: 0+j1
  note: Delayed alpha beta zero
  alpha_beta : Inport
  N_delay : Inport  Port=2
  wt : Inport  Port=3
  Alpha-Beta-Zero to dq0 : powerlib_meascontrol/Transformations/Alpha-Beta-Zero to dq0  Alignment=90 degrees behind phase A axis
      settings: SourceProductName=Simscape Power Systems
  Complex to Real-Imag : ComplexToRealImag
  Constant1 : Constant  Value=0
  Constant3 : Constant  Value=0
  Constant4 : Constant
  Demux : Demux  Outputs=2
  Demux1 : Demux  Outputs=2
  Gain : Gain  Gain=0.5
  Mux1 : Mux  Inputs=[1 1 1]
  Product : Product
  Real-Imag to Complex : RealImagToComplex
  Real-Imag to Complex1 : RealImagToComplex
  Real-Imag to Complex2 : RealImagToComplex
  Selector4 : Selector  InputPortWidth=3  IndexOptions=Index vector (dialog)  Indices=[1 2]  OutputSizes=1
  Subtract : Sum
  Variable Integer Delay : Delay  DelayLengthSource=Input port  DelayLength=200  DelayLengthUpperLimit=500  SampleTime=Ts
      settings: InputPortMap=u0,p1
  DSC_alpha_beta : Outport
  wires:
  Product/1 -> Subtract/2
  Demux/1 -> Real-Imag to Complex/1
  Real-Imag to Complex1/1 -> Product/1
  Demux1/1 -> Real-Imag to Complex1/1
  wt/1 -> Alpha-Beta-Zero to dq0/2
  Complex to Real-Imag/1 -> Mux1/1
  Variable Integer Delay/1 -> Demux1/1
  Demux1/2 -> Real-Imag to Complex1/2
  N_delay/1 -> Variable Integer Delay/2
  Gain/1 -> Alpha-Beta-Zero to dq0/1
  Constant3/1 -> Real-Imag to Complex2/1
  Real-Imag to Complex/1 -> Subtract/1
  alpha_beta/1 -> Variable Integer Delay/1, Demux/1
  Real-Imag to Complex2/1 -> Product/2
  Subtract/1 -> Complex to Real-Imag/1
  Constant1/1 -> Mux1/3
  Demux/2 -> Real-Imag to Complex/2
  Constant4/1 -> Real-Imag to Complex2/2
  Complex to Real-Imag/2 -> Mux1/2
  Mux1/1 -> Gain/1
  Alpha-Beta-Zero to dq0/1 -> Selector4/1
  Selector4/1 -> DSC_alpha_beta/1

== system pwrsys/Basic Blocks/DSC Power  ==
  valphabeta : Inport
  ialphabeta : Inport  Port=2
  Nsamp_delay : Inport  Port=3
  Complex to Real-Imag : ComplexToRealImag
  Complex to Real-Imag1 : ComplexToRealImag
  Constant3 : Constant  Value=0
  Constant4 : Constant
  Constant5 : Constant  Value=0
  Constant6 : Constant
  Demux{,2..3,5} (4 alike) : Demux  Outputs=2
  Gain : Gain  Gain=0.5
  Gain1 : Gain  Gain=0.5
  Mux1 : Mux  Inputs=[1 1]
  Mux2 : Mux  Inputs=[1 1]
  Product : Product
  Product1 : Product
  Real-Imag to Complex{,1..5} (6 alike) : RealImagToComplex
  Subtract : Sum
  Subtract1 : Sum
  Variable Integer Delay : Delay  DelayLengthSource=Input port  DelayLength=200  DelayLengthUpperLimit=500  SampleTime=Ts
      settings: InputPortMap=u0,p1
  Variable Integer Delay1 : Delay  DelayLengthSource=Input port  DelayLength=200  DelayLengthUpperLimit=500  SampleTime=Ts
      settings: InputPortMap=u0,p1
  valphabeta_DSC : Outport
  ialphabeta_DSC : Outport  Port=2
  wires:
  Demux2/2 -> Real-Imag to Complex1/2
  Demux3/1 -> Real-Imag to Complex3/1
  Constant6/1 -> Real-Imag to Complex5/2
  Constant5/1 -> Real-Imag to Complex5/1
  Real-Imag to Complex5/1 -> Product1/2
  Complex to Real-Imag1/1 -> Mux2/1
  Real-Imag to Complex4/1 -> Product1/1
  Demux3/2 -> Real-Imag to Complex3/2
  Gain1/1 -> ialphabeta_DSC/1  "ialphabeta"
  Complex to Real-Imag1/2 -> Mux2/2
  Complex to Real-Imag/1 -> Mux1/1
  Mux2/1 -> Gain1/1
  valphabeta/1 -> Demux/1, Variable Integer Delay/1
  Real-Imag to Complex2/1 -> Product/2
  Subtract1/1 -> Complex to Real-Imag1/1
  Real-Imag to Complex3/1 -> Subtract1/1
  Mux1/1 -> Gain/1
  Constant3/1 -> Real-Imag to Complex2/1
  Demux/1 -> Real-Imag to Complex/1
  Variable Integer Delay1/1 -> Demux5/1
  Demux5/2 -> Real-Imag to Complex4/2
  Demux2/1 -> Real-Imag to Complex1/1
  Variable Integer Delay/1 -> Demux2/1
  Product/1 -> Subtract/2
  Nsamp_delay/1 -> Variable Integer Delay1/2, Variable Integer Delay/2
  Complex to Real-Imag/2 -> Mux1/2
  Product1/1 -> Subtract1/2
  Gain/1 -> valphabeta_DSC/1  "valphabeta"
  Real-Imag to Complex1/1 -> Product/1
  Real-Imag to Complex/1 -> Subtract/1
  Subtract/1 -> Complex to Real-Imag/1
  Constant4/1 -> Real-Imag to Complex2/2
  ialphabeta/1 -> Demux3/1, Variable Integer Delay1/1
  Demux5/1 -> Real-Imag to Complex4/1
  Demux/2 -> Real-Imag to Complex/2

== system pwrsys/Basic Blocks/Digital first order LPF ==
  note: Transfer function: alpha / ( 1 + ( alpha -1 ) z^{-1} )
  note: alpha = Ts / ( 1/(2 pi fcutout) + Ts )
  note: y = alpha x + ( 1 - alpha) y z^{-1}
  in : Inport
  Add7 : Sum  Commented=on  Inputs=+-
  Discrete Filter : DiscreteFilter  Numerator=[Ts/(1/(2*pi*fcutout)+Ts)]  Denominator=[1 Ts/(1/(2*pi*fcutout)+Ts)-1]  SampleTime=Ts
  Discrete-Time Integrator : DiscreteIntegrator  Commented=on  IntegratorMethod=Integration: Trapezoidal  SampleTime=Ts  ICPrevOutput=DiscIntNeverNeededParam  ICPrevScaledInput=DiscIntNeverNeededParam
  Gain6 : Gain  Commented=on  Gain=2*pi*fcutout
  Rate Transition3 : RateTransition  OutPortSampleTime=Ts
  out : Outport
  wires:
  Add7/1 -> Gain6/1
  Discrete-Time Integrator/1 -> Add7/2
  in/1 -> Rate Transition3/1
  Gain6/1 -> Discrete-Time Integrator/1
  Rate Transition3/1 -> Add7/1, Discrete Filter/1
  Discrete Filter/1 -> out/1

== system pwrsys/Basic Blocks/Droop controller ==
  Delta : Inport
  Ref : Inport  Port=2
  Comp : Inport  Port=3
  Abs : Abs  ZeroCross=off
  Avoid div by zero : Sum
  Compensation : Product  Inputs=*/
  Constant : Constant  Value=1e-5
  Dead-band : DeadZone  LowerValue=-DB  UpperValue=DB  SaturateOnIntegerOverflow=on
  Low-pass filter : DiscreteIntegrator  gainval=flp  SampleTime=Ts  UpperSaturationLimit=Refmax/Kp  LowerSaturationLimit=Refmin/Kp  ICPrevOutput=DiscIntNeverNeededParam  ICPrevScaledInput=DiscIntNeverNeededParam
  Output Limit : Saturate  UpperLimit=Refmax  LowerLimit=Refmin  ZeroCross=off
  Permanent droop (Proportional) : Gain  Gain=Kp
  Relational Operator : RelationalOperator  Operator=~=  OutDataTypeStr=boolean  RndMeth=Simplest
  Reset time : Gain  Gain=1/Tr
  Setpoint Limit : Saturate  UpperLimit=Refmax  LowerLimit=Refmin  ZeroCross=off
  Sum1 : Sum  Inputs=--
  Sum2 : Sum
  Sum3 : Sum  Inputs=-+
  Sum6 : Sum  Inputs=-+
  Transient droop (Derivative) : Gain  Gain=Kd/Tr
  Washout filter : DiscreteIntegrator  gainval=1  ExternalReset=level  SampleTime=Ts  LimitOutput=on  UpperSaturationLimit=Refmax  LowerSaturationLimit=Refmin  ICPrevOutput=DiscIntNeverNeededParam  ICPrevScaledInput=DiscIntNeverNeededParam
  Out : Outport
  wires:
  Permanent droop (Proportional)/1 -> Sum1/2  "perm"
  Washout filter/1 -> Sum6/1
  Transient droop (Derivative)/1 -> Sum6/2
  Sum1/1 -> Sum2/1  "droop"
  Sum6/1 -> Sum1/1, Reset time/1  "trans"
  Reset time/1 -> Washout filter/1
  Sum2/1 -> Compensation/1  "outnc"
  Dead-band/1 -> Relational Operator/2, Permanent droop (Proportional)/1, Transient droop (Derivative)/1
  Setpoint Limit/1 -> Sum2/2  "reflim"
  Constant/1 -> Avoid div by zero/1
  Avoid div by zero/1 -> Compensation/2
  Output Limit/1 -> Out/1  "Out"
  Abs/1 -> Avoid div by zero/2
  Relational Operator/1 -> Washout filter/2
  Compensation/1 -> Output Limit/1  "outnl"
  Sum3/1 -> Low-pass filter/1
  Low-pass filter/1 -> Relational Operator/1, Sum3/1, Dead-band/1  "Delta_filt"
  Delta/1 -> Sum3/2
  Ref/1 -> Setpoint Limit/1
  Comp/1 -> Abs/1

== system pwrsys/Basic Blocks/PI controller with Hold ==
  Hold : Inport
  In : Inport  Port=2
  Anti-windup : Switch  Criteria=u2 ~= 0
  Discrete-Time Integrator : DiscreteIntegrator  InitialCondition=x0  SampleTime=Ts  UpperSaturationLimit=Max  LowerSaturationLimit=Min  ICPrevOutput=DiscIntNeverNeededParam  ICPrevScaledInput=DiscIntNeverNeededParam
  Eq. 10-X4 : Sum  SaturateOnIntegerOverflow=on  InputSameDT=on  OutDataTypeStr=Inherit: Same as first input
  Integral : Gain  Gain=Ki
  Logical Operator : Logic  Operator=OR  AllPortsSameDT=off  OutDataTypeStr=boolean
  Proportional : Gain  Gain=Kp
  Relational Operator : RelationalOperator  Operator=~=  OutDataTypeStr=boolean  RndMeth=Simplest
  Saturation : Saturate  UpperLimit=Max  LowerLimit=Min
  v1 : Constant  Value=0
  Out : Outport
  wires:
  Discrete-Time Integrator/1 -> Eq. 10-X4/2
  Integral/1 -> Anti-windup/3
  Anti-windup/1 -> Discrete-Time Integrator/1
  Hold/1 -> Logical Operator/1
  In/1 -> Integral/1, Proportional/1
  Eq. 10-X4/1 -> Saturation/1, Relational Operator/1
  v1/1 -> Anti-windup/1
  Saturation/1 -> Relational Operator/2, Out/1
  Logical Operator/1 -> Anti-windup/2
  Proportional/1 -> Eq. 10-X4/1
  Relational Operator/1 -> Logical Operator/2
